simulink model "PID"  (R2018b)
settings: Solver=VariableStepAuto  StartTime=0.0  StopTime=2  RelTol=1e-3
undefined symbols (not defined in the file): DIM, DIS, I1, I2, I3, M, magnitude
libraries: robotcorelib x5, simulink x3
settings Model: Creator=Paweł Tymiński  LastModifiedBy=Paweł Tymiński

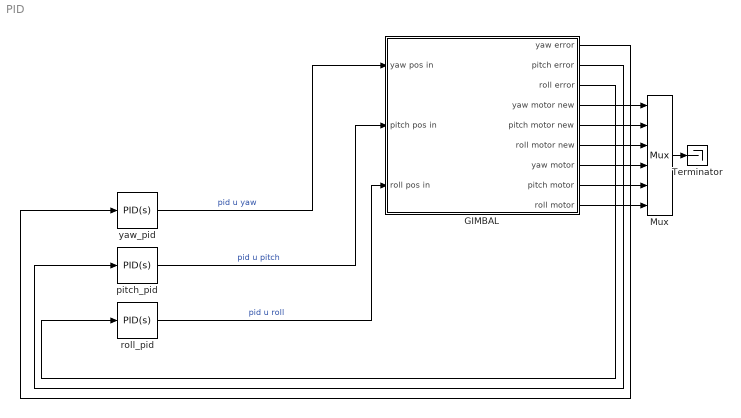
== system PID ==
  GIMBAL : Subsystem
  Mux : Mux  Inputs=6
  Terminator : Terminator
  pitch_pid : simulink/Continuous/PID Controller  Controller=PID  Form=Parallel  TimeDomain=Continuous-time  SampleTime=-1  IntegratorMethod=Forward Euler  FilterMethod=Forward Euler  ControllerParametersSource=internal  P=0.495  I=37  D=0.000775  UseFilter=on  N=100  TunerSelectOption=Transfer Function Based (PID Tuner App)  InitialConditionSource=internal  InitialConditionForIntegrator=0  InitialConditionForFilter=0  DifferentiatorICPrevScaledInput=0  ExternalReset=none  TrackingMode=off  Kt=1  LimitOutput=on  UpperSaturationLimit=inf  LowerSaturationLimit=-inf  LinearizeAsGain=on  AntiWindupMode=none  Kb=1  POutMin=[]  POutMax=[]  IOutMin=[]  IOutMax=[]  DOutMin=[]  DOutMax=[]  NOutMin=[]  NOutMax=[]  SumOutMin=[]  SumOutMax=[]  SaturationOutMin=[]  SaturationOutMax=[]  PParamMin=[]  PParamMax=[]  IParamMin=[]  IParamMax=[]  DParamMin=[]  DParamMax=[]  NParamMin=[]  NParamMax=[]  KbParamMin=[]  KbParamMax=[]  KtParamMin=[]  KtParamMax=[]  KbOutMin=[]  KbOutMax=[]  KtOutMin=[]  KtOutMax=[]  IntegratorOutMin=[]  IntegratorOutMax=[]  FilterOutMin=[]  FilterOutMax=[]  SumI1OutMin=[]  SumI1OutMax=[]  SumI2OutMin=[]  SumI2OutMax=[]  SumI3OutMin=[]  SumI3OutMax=[]  SumI4OutMin=[]  SumI4OutMax=[]  SumDOutMin=[]  SumDOutMax=[]  DifferentiatorOutMin=[]  DifferentiatorOutMax=[]  FilterDiffOutCoefMin=[]  FilterDiffOutCoefMax=[]  ReciprocalOutMin=[]  ReciprocalOutMax=[]  SumDenOutMin=[]  SumDenOutMax=[]  SumNumOutMin=[]  SumNumOutMax=[]  DivideOutMin=[]  DivideOutMax=[]  IntegratorContinuousStateAttributes=''  IntegratorStateMustResolveToSignalObject=off  IntegratorRTWStateStorageClass=Auto  FilterContinuousStateAttributes=''  FilterStateMustResolveToSignalObject=off  FilterRTWStateStorageClass=Auto  ParallelPVariant=InternalParameters  IdealPVariant=Disabled  IVariant=InternalParameters  DVariant=InternalParameters  IntegratorVariant=Continuous  SatVariant=Enabled  AWVariant=Passthrough  PCopyVariant=Disabled  TRVariant=Disabled  FdbkBlocksVariant=Forward  IdealPFdbkVariant=Disabled  SatFdbkVariant=Disabled  DerivativeFilterVariant=ContFilter  NVariant=InternalParameters  NCopyVariant=Disabled  FilterICVariant=InternalICsFilter  IntegratorICVariant=InternalICs  ExternalResetVariant=Disabled  TRSumVariant=Passthrough  SumFdbkVariant=Disabled  SumVariant=Sum_PID
  roll_pid : simulink/Continuous/PID Controller  Controller=PID  Form=Parallel  TimeDomain=Continuous-time  SampleTime=-1  IntegratorMethod=Forward Euler  FilterMethod=Forward Euler  ControllerParametersSource=internal  P=0.495  I=37  D=0.000775  UseFilter=on  N=100  TunerSelectOption=Transfer Function Based (PID Tuner App)  InitialConditionSource=internal  InitialConditionForIntegrator=0  InitialConditionForFilter=0  DifferentiatorICPrevScaledInput=0  ExternalReset=none  TrackingMode=off  Kt=1  LimitOutput=on  UpperSaturationLimit=inf  LowerSaturationLimit=-inf  LinearizeAsGain=on  AntiWindupMode=none  Kb=1  POutMin=[]  POutMax=[]  IOutMin=[]  IOutMax=[]  DOutMin=[]  DOutMax=[]  NOutMin=[]  NOutMax=[]  SumOutMin=[]  SumOutMax=[]  SaturationOutMin=[]  SaturationOutMax=[]  PParamMin=[]  PParamMax=[]  IParamMin=[]  IParamMax=[]  DParamMin=[]  DParamMax=[]  NParamMin=[]  NParamMax=[]  KbParamMin=[]  KbParamMax=[]  KtParamMin=[]  KtParamMax=[]  KbOutMin=[]  KbOutMax=[]  KtOutMin=[]  KtOutMax=[]  IntegratorOutMin=[]  IntegratorOutMax=[]  FilterOutMin=[]  FilterOutMax=[]  SumI1OutMin=[]  SumI1OutMax=[]  SumI2OutMin=[]  SumI2OutMax=[]  SumI3OutMin=[]  SumI3OutMax=[]  SumI4OutMin=[]  SumI4OutMax=[]  SumDOutMin=[]  SumDOutMax=[]  DifferentiatorOutMin=[]  DifferentiatorOutMax=[]  FilterDiffOutCoefMin=[]  FilterDiffOutCoefMax=[]  ReciprocalOutMin=[]  ReciprocalOutMax=[]  SumDenOutMin=[]  SumDenOutMax=[]  SumNumOutMin=[]  SumNumOutMax=[]  DivideOutMin=[]  DivideOutMax=[]  IntegratorContinuousStateAttributes=''  IntegratorStateMustResolveToSignalObject=off  IntegratorRTWStateStorageClass=Auto  FilterContinuousStateAttributes=''  FilterStateMustResolveToSignalObject=off  FilterRTWStateStorageClass=Auto  ParallelPVariant=InternalParameters  IdealPVariant=Disabled  IVariant=InternalParameters  DVariant=InternalParameters  IntegratorVariant=Continuous  SatVariant=Enabled  AWVariant=Passthrough  PCopyVariant=Disabled  TRVariant=Disabled  FdbkBlocksVariant=Forward  IdealPFdbkVariant=Disabled  SatFdbkVariant=Disabled  DerivativeFilterVariant=ContFilter  NVariant=InternalParameters  NCopyVariant=Disabled  FilterICVariant=InternalICsFilter  IntegratorICVariant=InternalICs  ExternalResetVariant=Disabled  TRSumVariant=Passthrough  SumFdbkVariant=Disabled  SumVariant=Sum_PID
  yaw_pid : simulink/Continuous/PID Controller  Controller=PID  Form=Parallel  TimeDomain=Continuous-time  SampleTime=-1  IntegratorMethod=Forward Euler  FilterMethod=Forward Euler  ControllerParametersSource=internal  P=0.495  I=37  D=0.000775  UseFilter=on  N=100  TunerSelectOption=Transfer Function Based (PID Tuner App)  InitialConditionSource=internal  InitialConditionForIntegrator=0  InitialConditionForFilter=0  DifferentiatorICPrevScaledInput=0  ExternalReset=none  TrackingMode=off  Kt=1  LimitOutput=on  UpperSaturationLimit=inf  LowerSaturationLimit=-inf  LinearizeAsGain=on  AntiWindupMode=none  Kb=1  POutMin=[]  POutMax=[]  IOutMin=[]  IOutMax=[]  DOutMin=[]  DOutMax=[]  NOutMin=[]  NOutMax=[]  SumOutMin=[]  SumOutMax=[]  SaturationOutMin=[]  SaturationOutMax=[]  PParamMin=[]  PParamMax=[]  IParamMin=[]  IParamMax=[]  DParamMin=[]  DParamMax=[]  NParamMin=[]  NParamMax=[]  KbParamMin=[]  KbParamMax=[]  KtParamMin=[]  KtParamMax=[]  KbOutMin=[]  KbOutMax=[]  KtOutMin=[]  KtOutMax=[]  IntegratorOutMin=[]  IntegratorOutMax=[]  FilterOutMin=[]  FilterOutMax=[]  SumI1OutMin=[]  SumI1OutMax=[]  SumI2OutMin=[]  SumI2OutMax=[]  SumI3OutMin=[]  SumI3OutMax=[]  SumI4OutMin=[]  SumI4OutMax=[]  SumDOutMin=[]  SumDOutMax=[]  DifferentiatorOutMin=[]  DifferentiatorOutMax=[]  FilterDiffOutCoefMin=[]  FilterDiffOutCoefMax=[]  ReciprocalOutMin=[]  ReciprocalOutMax=[]  SumDenOutMin=[]  SumDenOutMax=[]  SumNumOutMin=[]  SumNumOutMax=[]  DivideOutMin=[]  DivideOutMax=[]  IntegratorContinuousStateAttributes=''  IntegratorStateMustResolveToSignalObject=off  IntegratorRTWStateStorageClass=Auto  FilterContinuousStateAttributes=''  FilterStateMustResolveToSignalObject=off  FilterRTWStateStorageClass=Auto  ParallelPVariant=InternalParameters  IdealPVariant=Disabled  IVariant=InternalParameters  DVariant=InternalParameters  IntegratorVariant=Continuous  SatVariant=Enabled  AWVariant=Passthrough  PCopyVariant=Disabled  TRVariant=Disabled  FdbkBlocksVariant=Forward  IdealPFdbkVariant=Disabled  SatFdbkVariant=Disabled  DerivativeFilterVariant=ContFilter  NVariant=InternalParameters  NCopyVariant=Disabled  FilterICVariant=InternalICsFilter  IntegratorICVariant=InternalICs  ExternalResetVariant=Disabled  TRSumVariant=Passthrough  SumFdbkVariant=Disabled  SumVariant=Sum_PID
  wires:
  GIMBAL/2(pitch error) -> pitch_pid/1
  GIMBAL/3(roll error) -> roll_pid/1
  yaw_pid/1 -> GIMBAL/1(yaw pos in)  "pid u yaw"
  pitch_pid/1 -> GIMBAL/2(pitch pos in)  "pid u pitch"
  roll_pid/1 -> GIMBAL/3(roll pos in)  "pid u roll"
  GIMBAL/4(yaw motor new) -> Mux/1
  GIMBAL/5(pitch motor new) -> Mux/2
  GIMBAL/6(roll motor new) -> Mux/3
  GIMBAL/7(yaw motor) -> Mux/4
  GIMBAL/8(pitch motor) -> Mux/5
  GIMBAL/9(roll motor) -> Mux/6
  Mux/1 -> Terminator/1
  GIMBAL/1(yaw error) -> yaw_pid/1

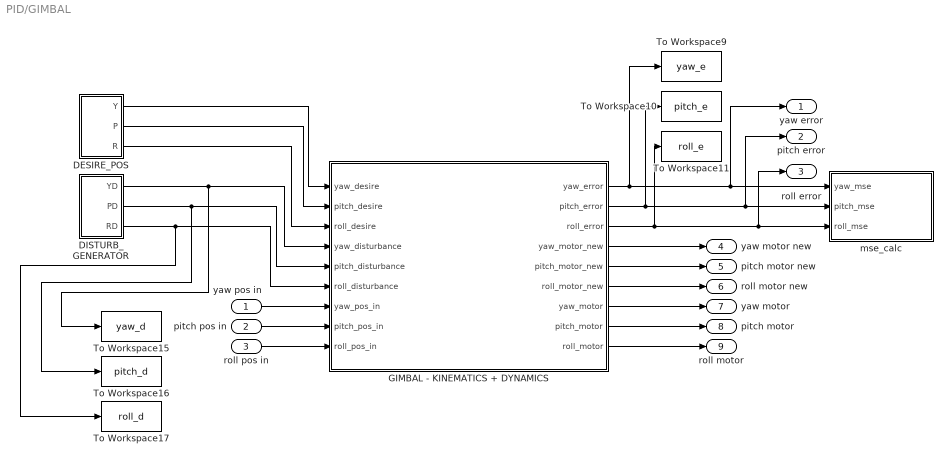
== system PID/GIMBAL ==
  yaw pos in : Inport
  pitch pos in : Inport  Port=2
  roll pos in : Inport  Port=3
  DESIRE_POS : Subsystem
  DISTURB_GENERATOR : Subsystem
  GIMBAL - KINEMATICS + DYNAMICS : Subsystem
  To Workspace10 : ToWorkspace  VariableName=pitch_e  SaveFormat=Timeseries  SampleTime=-1
  To Workspace11 : ToWorkspace  VariableName=roll_e  SaveFormat=Timeseries  SampleTime=-1
  To Workspace15 : ToWorkspace  VariableName=yaw_d  SaveFormat=Timeseries  SampleTime=-1
  To Workspace16 : ToWorkspace  VariableName=pitch_d  SaveFormat=Timeseries  SampleTime=-1
  To Workspace17 : ToWorkspace  VariableName=roll_d  SaveFormat=Timeseries  SampleTime=-1
  To Workspace9 : ToWorkspace  VariableName=yaw_e  SaveFormat=Timeseries  SampleTime=-1
  mse_calc : Subsystem
  yaw error : Outport
  pitch error : Outport  Port=2
  roll error : Outport  Port=3
  yaw motor new : Outport  Port=4
  pitch motor new : Outport  Port=5
  roll motor new : Outport  Port=6
  yaw motor : Outport  Port=7
  pitch motor : Outport  Port=8
  roll motor : Outport  Port=9
  wires:
  GIMBAL - KINEMATICS + DYNAMICS/9(roll_motor) -> roll motor/1
  GIMBAL - KINEMATICS + DYNAMICS/6(roll_motor_new) -> roll motor new/1
  GIMBAL - KINEMATICS + DYNAMICS/4(yaw_motor_new) -> yaw motor new/1
  yaw pos in/1 -> GIMBAL - KINEMATICS + DYNAMICS/7(yaw_pos_in)
  DESIRE_POS/3(R) -> GIMBAL - KINEMATICS + DYNAMICS/3(roll_desire)
  roll pos in/1 -> GIMBAL - KINEMATICS + DYNAMICS/9(roll_pos_in)
  GIMBAL - KINEMATICS + DYNAMICS/5(pitch_motor_new) -> pitch motor new/1
  GIMBAL - KINEMATICS + DYNAMICS/1(yaw_error) -> To Workspace9/1, yaw error/1, mse_calc/1(yaw_mse)
  GIMBAL - KINEMATICS + DYNAMICS/7(yaw_motor) -> yaw motor/1
  pitch pos in/1 -> GIMBAL - KINEMATICS + DYNAMICS/8(pitch_pos_in)
  DISTURB_GENERATOR/2(PD) -> To Workspace16/1, GIMBAL - KINEMATICS + DYNAMICS/5(pitch_disturbance)
  GIMBAL - KINEMATICS + DYNAMICS/3(roll_error) -> To Workspace11/1, roll error/1, mse_calc/3(roll_mse)
  DESIRE_POS/2(P) -> GIMBAL - KINEMATICS + DYNAMICS/2(pitch_desire)
  GIMBAL - KINEMATICS + DYNAMICS/2(pitch_error) -> To Workspace10/1, pitch error/1, mse_calc/2(pitch_mse)
  DISTURB_GENERATOR/3(RD) -> To Workspace17/1, GIMBAL - KINEMATICS + DYNAMICS/6(roll_disturbance)
  DESIRE_POS/1(Y) -> GIMBAL - KINEMATICS + DYNAMICS/1(yaw_desire)
  DISTURB_GENERATOR/1(YD) -> To Workspace15/1, GIMBAL - KINEMATICS + DYNAMICS/4(yaw_disturbance)
  GIMBAL - KINEMATICS + DYNAMICS/8(pitch_motor) -> pitch motor/1

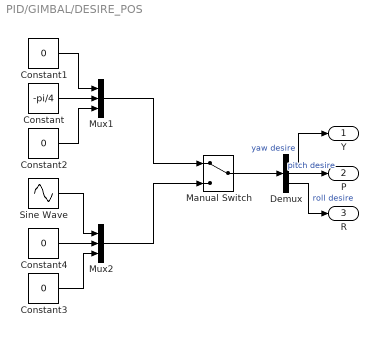
== system PID/GIMBAL/DESIRE_POS ==
  Constant : Constant  Value=-pi/4
  Constant{1..4} (4 alike) : Constant  Value=0
  Demux : Demux  Outputs=3
  Manual Switch : ManualSwitch
  Mux1 : Mux  Inputs=3
  Mux2 : Mux  Inputs=3
  Sine Wave : Sin  Amplitude=0.6  Frequency=0.25  SampleTime=0
  Y : Outport
  P : Outport  Port=2
  R : Outport  Port=3
  wires:
  Mux2/1 -> Manual Switch/2
  Constant4/1 -> Mux2/2
  Sine Wave/1 -> Mux2/1
  Constant2/1 -> Mux1/3
  Manual Switch/1 -> Demux/1
  Mux1/1 -> Manual Switch/1
  Constant1/1 -> Mux1/1
  Constant3/1 -> Mux2/3
  Constant/1 -> Mux1/2
  Demux/1 -> Y/1  "yaw desire"
  Demux/2 -> P/1  "pitch desire"
  Demux/3 -> R/1  "roll desire"

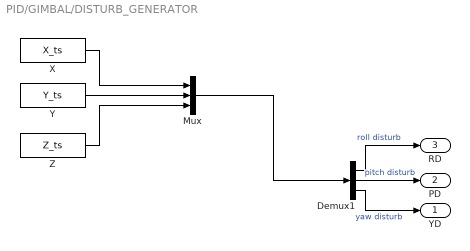
== system PID/GIMBAL/DISTURB_GENERATOR ==
  Demux1 : Demux  Outputs=3
  Mux : Mux  Inputs=3
  X : FromWorkspace  VariableName=X_ts  SampleTime=0.01  Interpolate=off  OutputAfterFinalValue=Setting to zero
  Y : FromWorkspace  VariableName=Y_ts  SampleTime=0.01  Interpolate=off  OutputAfterFinalValue=Setting to zero
  Z : FromWorkspace  VariableName=Z_ts  SampleTime=0.01  Interpolate=off  OutputAfterFinalValue=Setting to zero
  YD : Outport
  PD : Outport  Port=2
  RD : Outport  Port=3
  wires:
  X/1 -> Mux/1
  Y/1 -> Mux/2
  Z/1 -> Mux/3
  Demux1/3 -> YD/1  "yaw disturb"
  Mux/1 -> Demux1/1
  Demux1/1 -> RD/1  "roll disturb"
  Demux1/2 -> PD/1  "pitch disturb"

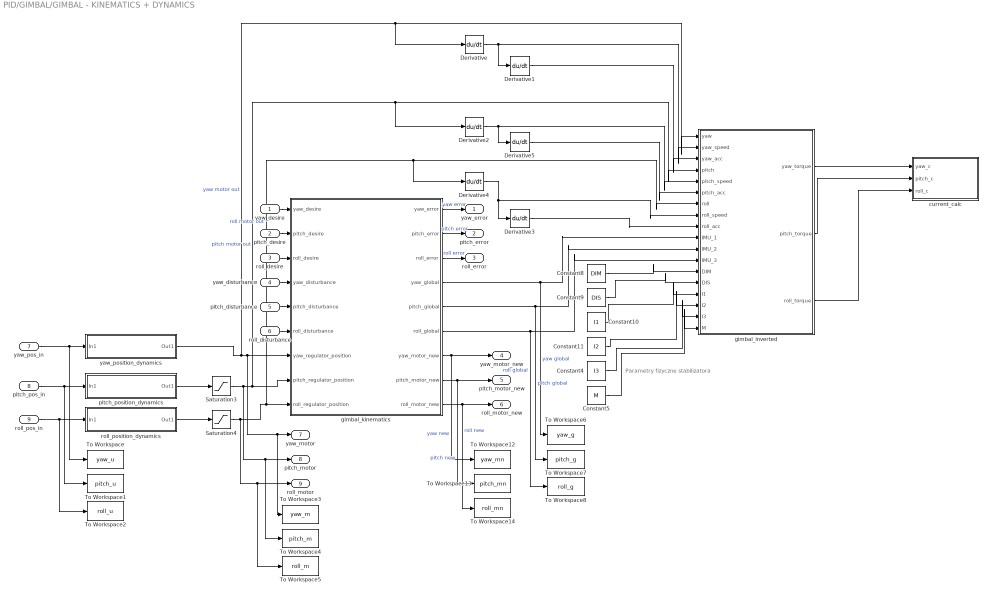
== system PID/GIMBAL/GIMBAL - KINEMATICS + DYNAMICS ==
  note: Parametry fizyczne stabilizatora
  yaw_desire : Inport
  pitch_desire : Inport  Port=2
  roll_desire : Inport  Port=3
  yaw_disturbance : Inport  Port=4
  pitch_disturbance : Inport  Port=5
  roll_disturbance : Inport  Port=6
  yaw_pos_in : Inport  Port=7
  pitch_pos_in : Inport  Port=8
  roll_pos_in : Inport  Port=9
  Constant10 : Constant  Value=I1
  Constant11 : Constant  Value=I2
  Constant4 : Constant  Value=I3
  Constant5 : Constant  Value=M
  Constant8 : Constant  Value=DIM
  Constant9 : Constant  Value=DIS
  Derivative{,1..5} (6 alike) : Derivative
  Saturation3 : Saturate  UpperLimit=2.35  LowerLimit=-2.35
  Saturation4 : Saturate  UpperLimit=0.78  LowerLimit=-0.78
  To Workspace : ToWorkspace  VariableName=yaw_u  SaveFormat=Timeseries  SampleTime=-1
  To Workspace1 : ToWorkspace  VariableName=pitch_u  SaveFormat=Timeseries  SampleTime=-1
  To Workspace12 : ToWorkspace  VariableName=yaw_mn  SaveFormat=Timeseries  SampleTime=-1
  To Workspace13 : ToWorkspace  VariableName=pitch_mn  SaveFormat=Timeseries  SampleTime=-1
  To Workspace14 : ToWorkspace  VariableName=roll_mn  SaveFormat=Timeseries  SampleTime=-1
  To Workspace2 : ToWorkspace  VariableName=roll_u  SaveFormat=Timeseries  SampleTime=-1
  To Workspace3 : ToWorkspace  VariableName=yaw_m  SaveFormat=Timeseries  SampleTime=-1
  To Workspace4 : ToWorkspace  VariableName=pitch_m  SaveFormat=Timeseries  SampleTime=-1
  To Workspace5 : ToWorkspace  VariableName=roll_m  SaveFormat=Timeseries  SampleTime=-1
  To Workspace6 : ToWorkspace  VariableName=yaw_g  SaveFormat=Timeseries  SampleTime=-1
  To Workspace7 : ToWorkspace  VariableName=pitch_g  SaveFormat=Timeseries  SampleTime=-1
  To Workspace8 : ToWorkspace  VariableName=roll_g  SaveFormat=Timeseries  SampleTime=-1
  current_calc : Subsystem
  gimbal_inverted : MATLAB Function  TreatAsAtomicUnit=on  SystemSampleTime=0.001
  gimbal_kinematics : Subsystem
  pitch_position_dynamics : Subsystem
  roll_position_dynamics : Subsystem
  yaw_position_dynamics : Subsystem
  yaw_error : Outport
  pitch_error : Outport  Port=2
  roll_error : Outport  Port=3
  yaw_motor_new : Outport  Port=4
  pitch_motor_new : Outport  Port=5
  roll_motor_new : Outport  Port=6
  yaw_motor : Outport  Port=7
  pitch_motor : Outport  Port=8
  roll_motor : Outport  Port=9
  wires:
  Constant9/1 -> gimbal_inverted/14(DIS)
  Derivative5/1 -> gimbal_inverted/6(pitch_acc)
  gimbal_kinematics/3(roll_error) -> roll_error/1  "roll error"
  pitch_desire/1 -> gimbal_kinematics/2(pitch_desire)
  yaw_position_dynamics/1(Out1) -> Derivative/1, gimbal_inverted/1(yaw), To Workspace3/1, yaw_motor/1, gimbal_kinematics/7(yaw_regulator_position)  "yaw motor out"
  gimbal_kinematics/9(roll_motor_new) -> To Workspace14/1, roll_motor_new/1  "roll new"
  Saturation4/1 -> To Workspace5/1, roll_motor/1, Derivative4/1, gimbal_inverted/7(roll), gimbal_kinematics/9(roll_regulator_position)  "roll motor out"
  roll_pos_in/1 -> To Workspace2/1, roll_position_dynamics/1(In1)
  Constant10/1 -> gimbal_inverted/15(I1)
  Derivative2/1 -> gimbal_inverted/5(pitch_speed), Derivative5/1
  gimbal_inverted/2(pitch_torque) -> current_calc/2(pitch_c)
  Derivative1/1 -> gimbal_inverted/3(yaw_acc)
  Constant11/1 -> gimbal_inverted/16(I2)
  roll_desire/1 -> gimbal_kinematics/3(roll_desire)
  yaw_disturbance/1 -> gimbal_kinematics/4(yaw_disturbance)
  Derivative/1 -> Derivative1/1, gimbal_inverted/2(yaw_speed)
  roll_position_dynamics/1(Out1) -> Saturation4/1
  Constant5/1 -> gimbal_inverted/18(M)
  gimbal_inverted/1(yaw_torque) -> current_calc/1(yaw_c)
  gimbal_kinematics/6(roll_global) -> To Workspace8/1, gimbal_inverted/12(IMU_3)  "roll global"
  Derivative4/1 -> Derivative3/1, gimbal_inverted/8(roll_speed)
  roll_disturbance/1 -> gimbal_kinematics/6(roll_disturbance)
  gimbal_inverted/3(roll_torque) -> current_calc/3(roll_c)
  gimbal_kinematics/7(yaw_motor_new) -> yaw_motor_new/1, To Workspace12/1  "yaw new"
  yaw_pos_in/1 -> To Workspace/1, yaw_position_dynamics/1(In1)
  Constant4/1 -> gimbal_inverted/17(I3)
  Constant8/1 -> gimbal_inverted/13(DIM)
  Saturation3/1 -> To Workspace4/1, pitch_motor/1, Derivative2/1, gimbal_inverted/4(pitch), gimbal_kinematics/8(pitch_regulator_position)  "pitch motor out"
  Derivative3/1 -> gimbal_inverted/9(roll_acc)
  pitch_position_dynamics/1(Out1) -> Saturation3/1
  gimbal_kinematics/5(pitch_global) -> To Workspace7/1, gimbal_inverted/11(IMU_2)  "pitch global"
  gimbal_kinematics/4(yaw_global) -> To Workspace6/1, gimbal_inverted/10(IMU_1)  "yaw global"
  gimbal_kinematics/1(yaw_error) -> yaw_error/1  "yaw error"
  pitch_disturbance/1 -> gimbal_kinematics/5(pitch_disturbance)
  gimbal_kinematics/2(pitch_error) -> pitch_error/1  "pitch error"
  gimbal_kinematics/8(pitch_motor_new) -> pitch_motor_new/1, To Workspace13/1  "pitch new"
  pitch_pos_in/1 -> To Workspace1/1, pitch_position_dynamics/1(In1)
  yaw_desire/1 -> gimbal_kinematics/1(yaw_desire)

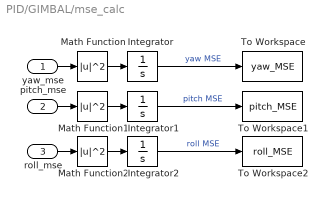
== system PID/GIMBAL/mse_calc ==
  yaw_mse : Inport
  pitch_mse : Inport  Port=2
  roll_mse : Inport  Port=3
  Integrator : Integrator
  Integrator1 : Integrator
  Integrator2 : Integrator
  Math Function : Math  Operator=magnitude^2  SaturateOnIntegerOverflow=on
  Math Function1 : Math  Operator=magnitude^2  SaturateOnIntegerOverflow=on
  Math Function2 : Math  Operator=magnitude^2  SaturateOnIntegerOverflow=on
  To Workspace : ToWorkspace  VariableName=yaw_MSE  SaveFormat=Timeseries  SampleTime=-1
  To Workspace1 : ToWorkspace  VariableName=pitch_MSE  SaveFormat=Timeseries  SampleTime=-1
  To Workspace2 : ToWorkspace  VariableName=roll_MSE  SaveFormat=Timeseries  SampleTime=-1
  wires:
  Integrator1/1 -> To Workspace1/1  "pitch MSE"
  Math Function2/1 -> Integrator2/1
  Integrator2/1 -> To Workspace2/1  "roll MSE"
  Math Function1/1 -> Integrator1/1
  yaw_mse/1 -> Math Function/1
  Math Function/1 -> Integrator/1
  roll_mse/1 -> Math Function2/1
  pitch_mse/1 -> Math Function1/1
  Integrator/1 -> To Workspace/1  "yaw MSE"

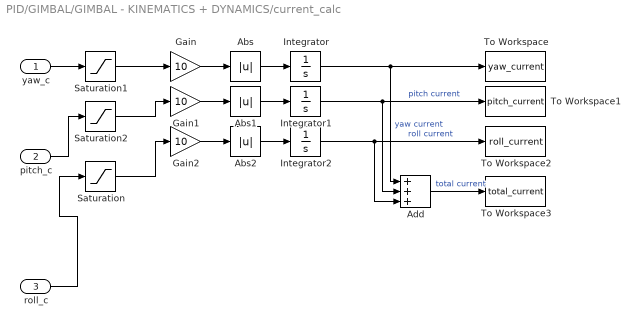
== system PID/GIMBAL/GIMBAL - KINEMATICS + DYNAMICS/current_calc ==
  yaw_c : Inport
  pitch_c : Inport  Port=2
  roll_c : Inport  Port=3
  Abs : Abs
  Abs1 : Abs
  Abs2 : Abs
  Add : Sum  Inputs=+++
  Gain : Gain  Gain=10
  Gain1 : Gain  Gain=10
  Gain2 : Gain  Gain=10
  Integrator : Integrator
  Integrator1 : Integrator
  Integrator2 : Integrator
  Saturation : Saturate  UpperLimit=0.34  LowerLimit=-0.34
  Saturation1 : Saturate  UpperLimit=0.34  LowerLimit=-.34
  Saturation2 : Saturate  UpperLimit=0.34  LowerLimit=-0.34
  To Workspace : ToWorkspace  VariableName=yaw_current  SaveFormat=Timeseries  SampleTime=-1
  To Workspace1 : ToWorkspace  VariableName=pitch_current  SaveFormat=Timeseries  SampleTime=-1
  To Workspace2 : ToWorkspace  VariableName=roll_current  SaveFormat=Timeseries  SampleTime=-1
  To Workspace3 : ToWorkspace  VariableName=total_current  SaveFormat=Timeseries  SampleTime=-1
  wires:
  Integrator1/1 -> Add/2, To Workspace1/1  "pitch current"
  Integrator/1 -> Add/1, To Workspace/1  "yaw current"
  Gain2/1 -> Abs2/1
  Gain/1 -> Abs/1
  Abs1/1 -> Integrator1/1
  Gain1/1 -> Abs1/1
  Abs2/1 -> Integrator2/1
  Abs/1 -> Integrator/1
  Saturation2/1 -> Gain1/1
  roll_c/1 -> Saturation/1
  Integrator2/1 -> Add/3, To Workspace2/1  "roll current"
  Saturation/1 -> Gain2/1
  Add/1 -> To Workspace3/1  "total current"
  Saturation1/1 -> Gain/1
  yaw_c/1 -> Saturation1/1
  pitch_c/1 -> Saturation2/1

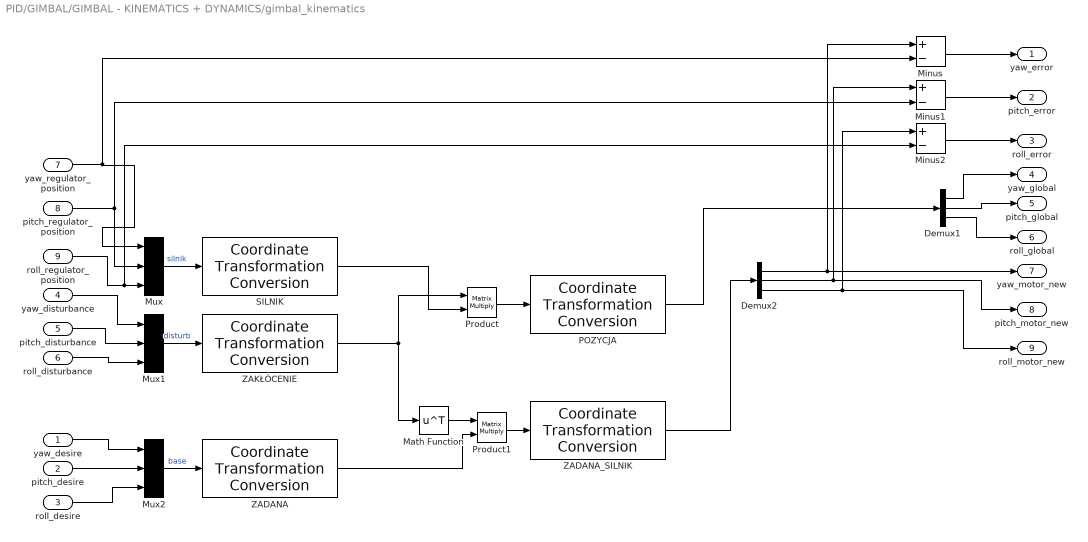
== system PID/GIMBAL/GIMBAL - KINEMATICS + DYNAMICS/gimbal_kinematics ==
  yaw_desire : Inport
  pitch_desire : Inport  Port=2
  roll_desire : Inport  Port=3
  yaw_disturbance : Inport  Port=4
  pitch_disturbance : Inport  Port=5
  roll_disturbance : Inport  Port=6
  yaw_regulator_position : Inport  Port=7
  pitch_regulator_position : Inport  Port=8
  roll_regulator_position : Inport  Port=9
  Demux1 : Demux  Outputs=3
  Demux2 : Demux  Outputs=3
  Math Function : Math  Operator=transpose  SaturateOnIntegerOverflow=on
  Minus : Sum  Inputs=+-
  Minus1 : Sum  Inputs=+-
  Minus2 : Sum  Inputs=+-
  Mux : Mux  Inputs=3
  Mux1 : Mux  Inputs=3
  Mux2 : Mux  Inputs=3
  POZYCJA : robotcorelib/Coordinate Transformation Conversion  InputRepresentation=Rotation Matrix  InputEulerSequence=ZYX  ShowTrVecInputPort=on  OutputRepresentation=Euler Angles  OutputEulerSequence=ZYX  ShowTrVecOutputPort=on  SimulateUsing=Interpreted execution
      settings: SourceProductBaseCode=RO
  Product : Product  Multiplication=Matrix(*)
  Product1 : Product  Multiplication=Matrix(*)
  SILNIK : robotcorelib/Coordinate Transformation Conversion  InputRepresentation=Euler Angles  InputEulerSequence=ZYX  ShowTrVecInputPort=on  OutputRepresentation=Rotation Matrix  OutputEulerSequence=ZYX  ShowTrVecOutputPort=on  SimulateUsing=Interpreted execution
      settings: SourceProductBaseCode=RO
  ZADANA : robotcorelib/Coordinate Transformation Conversion  InputRepresentation=Euler Angles  InputEulerSequence=ZYX  ShowTrVecInputPort=on  OutputRepresentation=Rotation Matrix  OutputEulerSequence=ZYX  ShowTrVecOutputPort=on  SimulateUsing=Interpreted execution
      settings: SourceProductBaseCode=RO
  ZADANA_SILNIK : robotcorelib/Coordinate Transformation Conversion  InputRepresentation=Rotation Matrix  InputEulerSequence=ZYX  ShowTrVecInputPort=on  OutputRepresentation=Euler Angles  OutputEulerSequence=ZYX  ShowTrVecOutputPort=on  SimulateUsing=Interpreted execution
      settings: SourceProductBaseCode=RO
  ZAKŁÓCENIE : robotcorelib/Coordinate Transformation Conversion  InputRepresentation=Euler Angles  InputEulerSequence=ZYX  ShowTrVecInputPort=on  OutputRepresentation=Rotation Matrix  OutputEulerSequence=ZYX  ShowTrVecOutputPort=on  SimulateUsing=Interpreted execution
      settings: SourceProductBaseCode=RO
  yaw_error : Outport
  pitch_error : Outport  Port=2
  roll_error : Outport  Port=3
  yaw_global : Outport  Port=4
  pitch_global : Outport  Port=5
  roll_global : Outport  Port=6
  yaw_motor_new : Outport  Port=7
  pitch_motor_new : Outport  Port=8
  roll_motor_new : Outport  Port=9
  wires:
  ZADANA_SILNIK/1 -> Demux2/1
  ZADANA/1 -> Product1/2
  Product/1 -> POZYCJA/1
  Mux1/1 -> ZAKŁÓCENIE/1  "disturb"
  SILNIK/1 -> Product/2
  Math Function/1 -> Product1/1
  Product1/1 -> ZADANA_SILNIK/1
  Mux/1 -> SILNIK/1  "silnik"
  Mux2/1 -> ZADANA/1  "base"
  ZAKŁÓCENIE/1 -> Math Function/1, Product/1
  pitch_desire/1 -> Mux2/2
  yaw_desire/1 -> Mux2/1
  roll_desire/1 -> Mux2/3
  yaw_disturbance/1 -> Mux1/1
  pitch_disturbance/1 -> Mux1/2
  roll_disturbance/1 -> Mux1/3
  roll_regulator_position/1 -> Mux/3, Minus2/2
  pitch_regulator_position/1 -> Mux/2, Minus1/2
  yaw_regulator_position/1 -> Mux/1, Minus/2
  Demux1/2 -> pitch_global/1
  Demux1/1 -> yaw_global/1
  Demux1/3 -> roll_global/1
  Demux2/1 -> Minus/1, yaw_motor_new/1
  Demux2/2 -> Minus1/1, pitch_motor_new/1
  Demux2/3 -> Minus2/1, roll_motor_new/1
  Minus/1 -> yaw_error/1
  POZYCJA/1 -> Demux1/1
  Minus1/1 -> pitch_error/1
  Minus2/1 -> roll_error/1

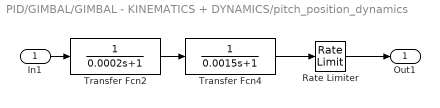
== system PID/GIMBAL/GIMBAL - KINEMATICS + DYNAMICS/pitch_position_dynamics ==
  In1 : Inport
  Rate Limiter : RateLimiter  RisingSlewLimit=18.5  FallingSlewLimit=-18.5  SampleTimeMode=inherited
  Transfer Fcn2 : TransferFcn  Denominator=[0.0002 1]
  Transfer Fcn4 : TransferFcn  Denominator=[0.0015 1]
  Out1 : Outport
  wires:
  Transfer Fcn2/1 -> Transfer Fcn4/1
  In1/1 -> Transfer Fcn2/1
  Transfer Fcn4/1 -> Rate Limiter/1
  Rate Limiter/1 -> Out1/1

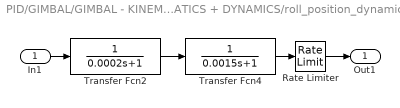
== system PID/GIMBAL/GIMBAL - KINEMATICS + DYNAMICS/roll_position_dynamics ==
  In1 : Inport
  Rate Limiter : RateLimiter  RisingSlewLimit=18.5  FallingSlewLimit=-18.5  SampleTimeMode=inherited
  Transfer Fcn2 : TransferFcn  Denominator=[0.0002 1]
  Transfer Fcn4 : TransferFcn  Denominator=[0.0015 1]
  Out1 : Outport
  wires:
  Transfer Fcn2/1 -> Transfer Fcn4/1
  In1/1 -> Transfer Fcn2/1
  Transfer Fcn4/1 -> Rate Limiter/1
  Rate Limiter/1 -> Out1/1

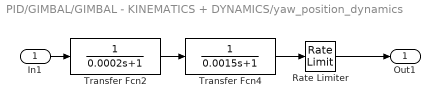
== system PID/GIMBAL/GIMBAL - KINEMATICS + DYNAMICS/yaw_position_dynamics ==
  In1 : Inport
  Rate Limiter : RateLimiter  RisingSlewLimit=18.5  FallingSlewLimit=-18.5  SampleTimeMode=inherited
  Transfer Fcn2 : TransferFcn  Denominator=[0.0002 1]
  Transfer Fcn4 : TransferFcn  Denominator=[0.0015 1]
  Out1 : Outport
  wires:
  Transfer Fcn2/1 -> Transfer Fcn4/1
  In1/1 -> Transfer Fcn2/1
  Transfer Fcn4/1 -> Rate Limiter/1
  Rate Limiter/1 -> Out1/1

== matlab function PID/GIMBAL/GIMBAL - KINEMATICS + DYNAMICS/gimbal_inverted ==
  data: yaw input; yaw_speed input; yaw_acc input; pitch input; pitch_speed input; pitch_acc input; roll input; yaw_torque output; roll_speed input; roll_acc input; IMU_1 input; IMU_2 input; IMU_3 input; DIM input; DIS input; I1 input; I2 input; I3 input; M input; pitch_torque output; roll_torque output
function [yaw_torque, pitch_torque, roll_torque]  = gimbal_dynamics(yaw,yaw_speed,yaw_acc,pitch,pitch_speed,pitch_acc,roll,roll_speed, roll_acc,IMU_1,IMU_2,IMU_3,DIM,DIS,I1,I2,I3,M)

%stała grawitacji
g = 9.81;


%-------------ZMIENNE--------------
% odczyty z IMU
alpha_1 = IMU_1;
alpha_2 = IMU_2;
alpha_3 = IMU_3;
IMU = [alpha_1; alpha_2; alpha_3];
%predkosci katowe osiagane przez gimbal
 om_1 = yaw_speed ;
 om_2 = pitch_speed ;
 om_3 = roll_speed ;
Omega = [om_1; om_2; om_3];
%kąty osiagane aktualnie przez gimbal
 theta_1 = yaw ;
 theta_2 = pitch ;
 theta_3 = roll ;
 THETA = [theta_1; theta_2; theta_3];
% przyśpieszenia kątowe w osiach gimbala
 ACC = [yaw_acc;pitch_acc;roll_acc];

%---------------FUNKCJE---------------------

H = calculate_H_matrix(THETA,Omega,I1,I2,I3,DIM);
D = calculate_D_matrix(THETA,I1,I2,I3,DIM);
G = calculate_G_matrix(IMU,THETA,DIM,M,DIS);
Q = D*ACC+H+G;
yaw_torque = Q(1);
pitch_torque = Q(2);
roll_torque = Q(3);

end
